simulink subsystem "O2_dissociation_inv"  (R2020b)
settings: Solver=VariableStepAuto  StartTime=0.0  StopTime=10.0  RelTol=1e-3
settings Model: Creator=RH  LastModifiedBy=Marco

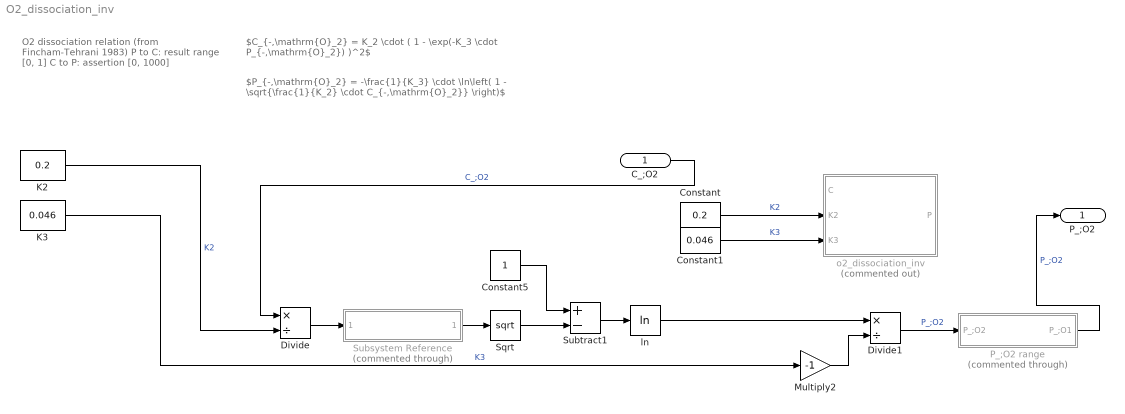
== system O2_dissociation_inv ==
  note: O2 dissociation relation
      | (from Fincham-Tehrani 1983)
      |
      | P to C: result range [0, 1]
      | C to P: assertion [0, 1000]
  note: $C_{-,\mathrm{O}_2} = K_2 \cdot ( 1 - \exp(-K_3 \cdot P_{-,\mathrm{O}_2}) )^2$
  note: $P_{-,\mathrm{O}_2} = -\frac{1}{K_3} \cdot \ln\left( 1 - \sqrt{\frac{1}{K_2} \cdot C_{-,\mathrm{O}_2}} \right)$
  C_;O2 : Inport  Unit=1
  Constant : Constant  Value=0.2
  Constant1 : Constant  Value=0.046
  Constant5 : Constant
  Divide : Product  Inputs=*/
  Divide1 : Product  Inputs=*/
  K2 : Constant  Value=0.2
  K3 : Constant  Value=0.046
  Multiply2 : Gain  Gain=-1
  P_;O2 range : Subsystem  Commented=through
  Sqrt : Sqrt  SaturateOnIntegerOverflow=on
  Subsystem Reference : Subsystem  Commented=through  ReferencedSubsystem=saturation_range
  Subtract1 : Sum  Inputs=+-
  ln : Math  Operator=log  SaturateOnIntegerOverflow=on
  o2_dissociation_inv : MATLAB Function  Commented=on  TreatAsAtomicUnit=on
  P_;O2 : Outport  Unit=mmHg
  wires:
  Subtract1/1 -> ln/1
  Divide/1 -> Subsystem Reference/1
  Multiply2/1 -> Divide1/2
  Constant5/1 -> Subtract1/1
  K3/1 -> Multiply2/1  "K3"
  K2/1 -> Divide/2  "K2"
  Sqrt/1 -> Subtract1/2
  Subsystem Reference/1 -> Sqrt/1
  ln/1 -> Divide1/1
  Divide1/1 -> P_;O2 range/1(P_;O2)  "P_;O2"
  Constant/1 -> o2_dissociation_inv/2(K2)  "K2"
  Constant1/1 -> o2_dissociation_inv/3(K3)  "K3"
  C_;O2/1 -> Divide/1  "C_;O2"
  P_;O2 range/1(P_;O1) -> P_;O2/1  "P_;O2"

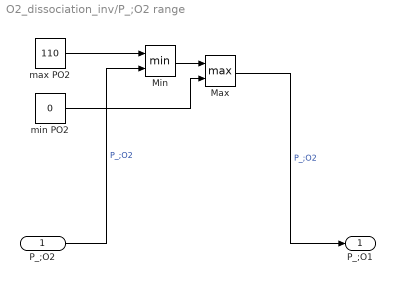
== system O2_dissociation_inv/P_;O2 range ==
  P_;O2 : Inport
  Max : MinMax  Function=max  Inputs=2
  Min : MinMax  Inputs=2
  max PO2 : Constant  Value=110
  min PO2 : Constant  Value=0
  P_;O1 : Outport
  wires:
  P_;O2/1 -> Min/2  "P_;O2"
  min PO2/1 -> Max/2
  Min/1 -> Max/1
  max PO2/1 -> Min/1
  Max/1 -> P_;O1/1  "P_;O2"

== matlab function O2_dissociation_inv/o2_dissociation_inv ==
  data: C input; P output; K2 input; K3 input
function P = o2_dissociation_inv(C, K2, K3)
    d = 0.0001;
%     m = 1000;
%     pmax = 125;
    cmax = K2 - d;
%     pmax = -1/K3 * log(1-sqrt(K2 * (1-d)));
    C = min(C, cmax);
    C = max(0, C);
    P = -1/K3 * log(1-sqrt(1/K2 * C));
%     if C < K2 - d
%         P = -1/K3 * log(1-sqrt(1/K2 * C));
%     else
% %         P = pmax;
% %         P = -1/K3 * log(1-sqrt(K2 * (1-d))) + (C-(K2-d))*m;
%         P = pmax;
%     end
end
